simulink model "questao2_3"  (R2024b)
settings: Solver=VariableStepAuto  StartTime=0.0  StopTime=20  RelTol=1e-3
libraries: cstblocks x1
settings Model: Creator=bruno  LastModifiedBy=bruno

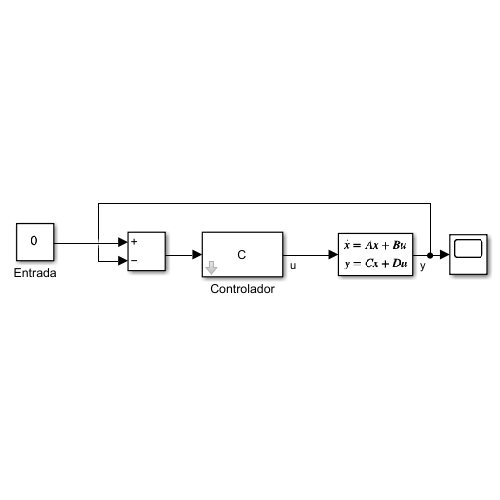
[thumbnail: Simulink's stored preview of the top-level diagram]
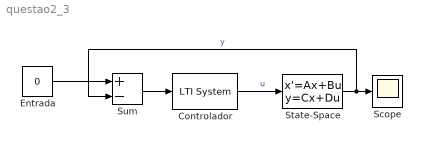
== system questao2_3 ==
  Controlador : cstblocks/LTI System  sys=C  IC=[]  PadeOrder=0
  Entrada : Constant  Value=0
  Scope : Scope
  State-Space : StateSpace  A=|  B=[0; 0; 0.6667; 0.6667]  C=[0, 1, 0, 0]  D=0  InitialCondition=0.174533
      | [0,     0,     1,     0;
      |      0,     0,     0,     1;
      |      0,  3.273, -0.006667, -0.006667;  0, 13.09,  -0.006667,  -0.02667]
  Sum : Sum  Inputs=+-
  wires:
  Sum/1 -> Controlador/1
  Controlador/1 -> State-Space/1  "u"
  Entrada/1 -> Sum/1
  State-Space/1 -> Sum/2, Scope/1  "y"
